simulink model "RETE_NORMALE_DEFINITIVA"  (R2024a)
settings: Solver=VariableStepAuto  StartTime=0.0  StopTime=9000  RelTol=1e-3
libraries: fl_lib x31, nesl_utility x8, simulink x2
(part 2 of 2)

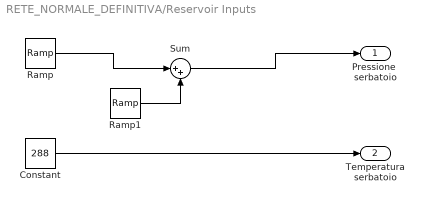
== system RETE_NORMALE_DEFINITIVA/Reservoir Inputs ==
  Constant : Constant  Value=288
  Ramp : simulink/Sources/Ramp  slope=-0.1  start=3  InitialOutput=7.4
  Ramp1 : simulink/Sources/Ramp  slope=0.1  start=5  InitialOutput=0
  Sum : Sum  Inputs=|++
  Pressione  serbatoio : Outport
  Temperatura serbatoio : Outport  Port=2
  wires:
  Constant/1 -> Temperatura serbatoio/1
  Ramp/1 -> Sum/1
  Sum/1 -> Pressione  serbatoio/1
  Ramp1/1 -> Sum/2
